simulink model "mcb_pmsm_foc_dual_cpu1_f28379d"  (R2024b)
settings: Solver=FixedStepDiscrete  StartTime=0.0  StopTime=6  RelTol=1e-3  EnableMultiTasking=on
InitFcn:
  | mcb_pmsm_foc_dual_f28379d_datascript;
model workspace (MAT data in the model file):
  encoderResolution = 2000
  hallOffset = '0.5'
  indexOffset = 850
  polePairs = '4'
values from neighbouring files (symbols this model uses):
  acceleration = 20000/PU_System_motor1.N_base    [mcb_pmsm_foc_sensorless_dyno_f28379d_datascript.m]    (also in soc_mcb_pmsm_foc_dyno_f28379d_data.m = 20000/PU_System.N_base)
  dataType = 'single'    [mcb_pmsm_foc_sensorless_dyno_f28379d_datascript.m]    (also in soc_mcb_pmsm_foc_dyno_f28379d_data.m)
  inverter = mcb_SetInverterParameters('BoostXL-DRV8305')    [soc_mcb_pmsm_foc_dyno_f28379d_data.m]
  Speed_openLoop_PU = 0.1    [mcb_pmsm_foc_sensorless_dyno_f28379d_datascript.m]    (also in soc_mcb_pmsm_foc_dyno_f28379d_data.m)
  target = mcb_SetProcessorDetails('F28379D',PWM_frequency)    [mcb_pmsm_foc_sensorless_dyno_f28379d_datascript.m]    (also in soc_mcb_pmsm_foc_dyno_f28379d_data.m)
  Ts = T_pwm    (= 5e-05)    [mcb_pmsm_foc_sensorless_dyno_f28379d_datascript.m]    (also in soc_mcb_pmsm_foc_dyno_f28379d_data.m)
  Ts_speed = 20*Ts    (= 0.001)    [mcb_pmsm_foc_sensorless_dyno_f28379d_datascript.m]    (also in soc_mcb_pmsm_foc_dyno_f28379d_data.m)
undefined symbols (not defined in the file or in its folder): Down, GPTRIP1SEL, GPTRIP2SEL, TZ1, TZ2, Up
libraries: c2802xlib x9, c2837xDlib x5, procinterlib x4, simulink x3, c280xlib x3, demo_controls x1, svdschedulerlib x1, mcbpmsmnonlinearlib x1, svdutilitieslib x1
(part 2 of 2)

== system mcb_pmsm_foc_dual_cpu1_f28379d/Serial Receive/Data Receive/Data_Type_Float ==
  SCI Receive : c280xlib/SCI Receive  sciModule=A  dataHead=''  headerCheckMaxCount=16  dataTail=''  dataType=single  dataLenOptions=Length via dialog  dataDim=4  maxDataLength=1  initValue=0  errOption=Output the last received value  errValue=0  sampleTime=-1  blockingMode=on  timeOut=0.00875  outputStatus=off
  Out1 : Outport
  wires:
  SCI Receive/1 -> Out1/1

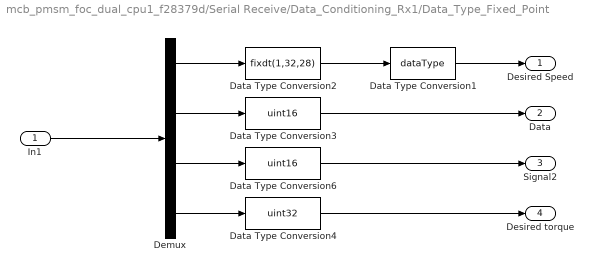
== system mcb_pmsm_foc_dual_cpu1_f28379d/Serial Receive/Data_Conditioning_Rx1/Data_Type_Fixed_Point ==
  In1 : Inport
  Data Type Conversion1 : DataTypeConversion  OutDataTypeStr=dataType  RndMeth=Simplest  SaturateOnIntegerOverflow=off
  Data Type Conversion2 : DataTypeConversion  OutDataTypeStr=fixdt(1,32,28)  ConvertRealWorld=Stored Integer (SI)  RndMeth=Simplest  SaturateOnIntegerOverflow=off
  Data Type Conversion3 : DataTypeConversion  OutDataTypeStr=uint16  RndMeth=Simplest  SaturateOnIntegerOverflow=off
  Data Type Conversion4 : DataTypeConversion  OutDataTypeStr=uint32  RndMeth=Simplest  SaturateOnIntegerOverflow=off
  Data Type Conversion6 : DataTypeConversion  OutDataTypeStr=uint16  RndMeth=Simplest  SaturateOnIntegerOverflow=off
  Demux : Demux
  Desired Speed : Outport
  Data : Outport  Port=2
  Signal2 : Outport  Port=3
  Desired torque : Outport  Port=4
  wires:
  In1/1 -> Demux/1
  Data Type Conversion1/1 -> Desired Speed/1
  Data Type Conversion2/1 -> Data Type Conversion1/1
  Demux/1 -> Data Type Conversion2/1
  Demux/2 -> Data Type Conversion3/1
  Data Type Conversion3/1 -> Data/1
  Demux/4 -> Data Type Conversion4/1
  Demux/3 -> Data Type Conversion6/1
  Data Type Conversion6/1 -> Signal2/1
  Data Type Conversion4/1 -> Desired torque/1

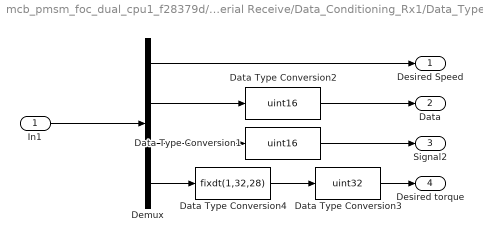
== system mcb_pmsm_foc_dual_cpu1_f28379d/Serial Receive/Data_Conditioning_Rx1/Data_Type_Float ==
  In1 : Inport
  Data Type Conversion1 : DataTypeConversion  OutDataTypeStr=uint16  RndMeth=Simplest  SaturateOnIntegerOverflow=off
  Data Type Conversion2 : DataTypeConversion  OutDataTypeStr=uint16  RndMeth=Simplest  SaturateOnIntegerOverflow=off
  Data Type Conversion3 : DataTypeConversion  OutDataTypeStr=uint32  ConvertRealWorld=Stored Integer (SI)  RndMeth=Simplest  SaturateOnIntegerOverflow=off
  Data Type Conversion4 : DataTypeConversion  OutDataTypeStr=fixdt(1,32,28)  RndMeth=Simplest  SaturateOnIntegerOverflow=off
  Demux : Demux
  Desired Speed : Outport
  Data : Outport  Port=2
  Signal2 : Outport  Port=3
  Desired torque : Outport  Port=4
  wires:
  In1/1 -> Demux/1
  Demux/1 -> Desired Speed/1
  Data Type Conversion2/1 -> Data/1
  Demux/2 -> Data Type Conversion2/1
  Demux/3 -> Data Type Conversion1/1
  Demux/4 -> Data Type Conversion4/1
  Data Type Conversion1/1 -> Signal2/1
  Data Type Conversion3/1 -> Desired torque/1
  Data Type Conversion4/1 -> Data Type Conversion3/1

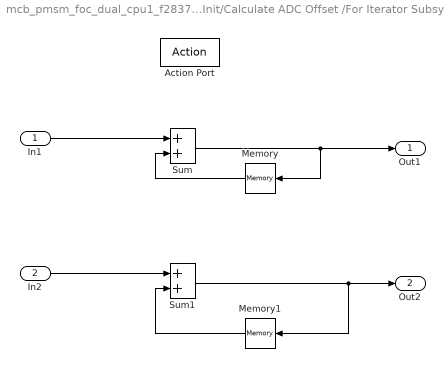
== system mcb_pmsm_foc_dual_cpu1_f28379d/Hardware Init/Calculate ADC Offset /For Iterator Subsystem/If Action Subsystem ==
  In1 : Inport
  In2 : Inport  Port=2
  Action Port : ActionPort  ActionPortLabel=if(u1 > 8)
  Memory : Memory  InheritSampleTime=on
  Memory1 : Memory  InheritSampleTime=on
  Sum : Sum
  Sum1 : Sum
  Out1 : Outport
  Out2 : Outport  Port=2
  wires:
  In1/1 -> Sum/1
  Sum/1 -> Out1/1, Memory/1
  In2/1 -> Sum1/1
  Memory/1 -> Sum/2
  Sum1/1 -> Out2/1, Memory1/1
  Memory1/1 -> Sum1/2

== system mcb_pmsm_foc_dual_cpu1_f28379d/Inverter Driver Peripherals/SCI Data Transmission/Data_Conditioning_Tx/Data_Type_Fixed_Point ==
  In1 : Inport
  Data Type Conversion : DataTypeConversion  OutDataTypeStr=fixdt(1,32,28)  RndMeth=Simplest  SaturateOnIntegerOverflow=off
  Data Type Conversion3 : DataTypeConversion  OutDataTypeStr=uint32  ConvertRealWorld=Stored Integer (SI)  RndMeth=Simplest  SaturateOnIntegerOverflow=off
  Data_Log : Outport
  wires:
  In1/1 -> Data Type Conversion/1
  Data Type Conversion3/1 -> Data_Log/1
  Data Type Conversion/1 -> Data Type Conversion3/1

== system mcb_pmsm_foc_dual_cpu1_f28379d/Inverter Driver Peripherals/SCI Data Transmission/Data_Conditioning_Tx/Data_Type_Float ==
  In1 : Inport
  Byte Pack : svdutilitieslib/Byte Pack  maskPackedDataType=uint32  datatypes={'single'}  byteAlign=4  blockPlatform=tic2000
  Data_Log : Outport
  wires:
  Byte Pack/1 -> Data_Log/1
  In1/1 -> Byte Pack/1

== system mcb_pmsm_foc_dual_cpu1_f28379d/Inverter Driver Peripherals/SCI Data Transmission/Data_Logging/Data ==
  Data : Inport
  Data_width : Inport  Port=2
  Action Port : ActionPort  ActionPortLabel=else
  Dummy : Constant  Value=hex2dec('0000')  OutDataTypeStr=uint32
  Mux : Mux  Inputs=2
  Data_out : Outport  VectorParamsAs1DForOutWhenUnconnected=off
  Iteration : Outport  Port=2  VectorParamsAs1DForOutWhenUnconnected=off
  wires:
  Data_width/1 -> Iteration/1
  Data/1 -> Mux/1
  Dummy/1 -> Mux/2
  Mux/1 -> Data_out/1

== system mcb_pmsm_foc_dual_cpu1_f28379d/Inverter Driver Peripherals/SCI Data Transmission/Data_Logging/End ==
  Data : Inport
  Data_width : Inport  Port=2
  Action Port : ActionPort  ActionPortLabel=elseif(u1 == 599)
  Bias : Bias  Bias=1  SaturateOnIntegerOverflow=off
  End : Constant  Value=hex2dec('45454545')  OutDataTypeStr=uint32
  Mux : Mux  Inputs=2
  Data_out : Outport  VectorParamsAs1DForOutWhenUnconnected=off
  Iteration : Outport  Port=2  VectorParamsAs1DForOutWhenUnconnected=off
  wires:
  Data/1 -> Mux/1
  Data_width/1 -> Bias/1
  Bias/1 -> Iteration/1
  End/1 -> Mux/2
  Mux/1 -> Data_out/1

== system mcb_pmsm_foc_dual_cpu1_f28379d/Inverter Driver Peripherals/SCI Data Transmission/Data_Logging/Start ==
  Data : Inport
  Data_width : Inport  Port=2
  Action Port : ActionPort  ActionPortLabel=if(u1 == 0)
  Bias : Bias  Bias=1  SaturateOnIntegerOverflow=off
  Mux : Mux  Inputs=2
  Start : Constant  Value=hex2dec('53535353')  OutDataTypeStr=uint32
  Data_out : Outport  VectorParamsAs1DForOutWhenUnconnected=off
  Iteration : Outport  Port=2  VectorParamsAs1DForOutWhenUnconnected=off
  wires:
  Data/1 -> Mux/2
  Data_width/1 -> Bias/1
  Bias/1 -> Iteration/1
  Start/1 -> Mux/1
  Mux/1 -> Data_out/1
